simulink model "es2s"  (R2020b)
settings: Solver=VariableStepAuto  StartTime=0.0  StopTime=20  MaxStep=0.001  RelTol=1e-3
values from neighbouring files (symbols this model uses):
  c = 0    [ex 5 residual solution.m]
  k = 100    [ex 5 residual solution.m]
  m = 2    [ex 5 residual solution.m]
undefined symbols (not defined in the file or in its folder): sigbuilder_block
settings Model: Creator=EREN  LastModifiedBy=drart

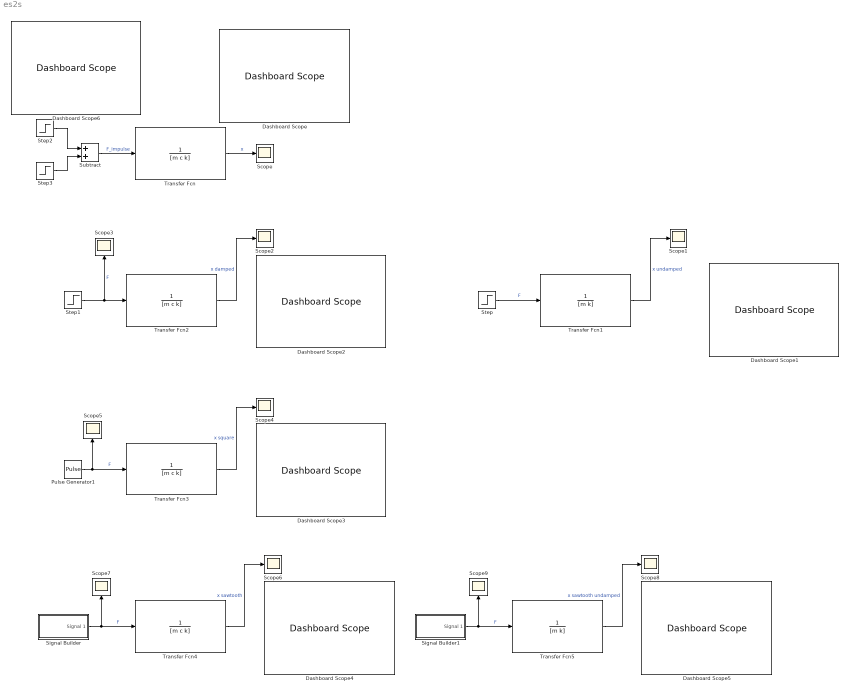
== system es2s ==
  Dashboard Scope{,1..6} (7 alike) : DashboardScope
  Pulse Generator1 : DiscretePulseGenerator  PulseType=Time based  Amplitude=50  Period=100  PulseWidth=5
  Scope{,1..9} (10 alike) : Scope
  Signal Builder : Subsystem  Tag=STV Subsys  LoadFcn=sigbuilder_block('load');  StartFcn=sigbuilder_block('start');  StopFcn=sigbuilder_block('stop');  ClipboardFcn=sigbuilder_block('clipboard');  mask(Sigbuilder block){tuvar=[0:10]}
      mask help: Simulink:masks:SigbuilderBlock_MD
      mask init:
      | if ~strcmp(get_param(bdroot(gcbh),'SimulationStatus'),'stopped') tuvar = sigbuilder_block('maskInit'); end
      settings: CopyFcn=sigbuilder_block('copy');  DeleteFcn=sigbuilder_block('delete');  ModelCloseFcn=sigbuilder_block('modelClose');  PreSaveFcn=sigbuilder_block('preSave');  PauseFcn=sigbuilder_block('pause');  ContinueFcn=sigbuilder_block('continue');  NameChangeFcn=sigbuilder_block('namechange');  OpenFcn=sigbuilder_block('open',[374.4 130.2 550.8 400.2 ]);  CloseFcn=sigbuilder_block('close');
      mask Display: plot(0, 0, 100, 100,[2, 2, 32, 32, 2], [68, 8, 8, 68, 68],[32, 2], [38, 38], [32, 19, 2],[53, 60, 44], [32, 17, 17, 2],[16, 16, 31, 31]);txt = getActiveGroup(gcbh);text(2, 100, txt,'verticalAlignment', 'top');
  Signal Builder1 : Subsystem  Tag=STV Subsys  LoadFcn=sigbuilder_block('load');  StartFcn=sigbuilder_block('start');  StopFcn=sigbuilder_block('stop');  ClipboardFcn=sigbuilder_block('clipboard');  mask(Sigbuilder block){tuvar=[0:10]}
      mask help: Simulink:masks:SigbuilderBlock_MD
      mask init:
      | if ~strcmp(get_param(bdroot(gcbh),'SimulationStatus'),'stopped') tuvar = sigbuilder_block('maskInit'); end
      settings: CopyFcn=sigbuilder_block('copy');  DeleteFcn=sigbuilder_block('delete');  ModelCloseFcn=sigbuilder_block('modelClose');  PreSaveFcn=sigbuilder_block('preSave');  PauseFcn=sigbuilder_block('pause');  ContinueFcn=sigbuilder_block('continue');  NameChangeFcn=sigbuilder_block('namechange');  OpenFcn=sigbuilder_block('open',[374.4 130.2 550.8 400.2 ]);  CloseFcn=sigbuilder_block('close');
      mask Display: plot(0, 0, 100, 100,[2, 2, 32, 32, 2], [68, 8, 8, 68, 68],[32, 2], [38, 38], [32, 19, 2],[53, 60, 44], [32, 17, 17, 2],[16, 16, 31, 31]);txt = getActiveGroup(gcbh);text(2, 100, txt,'verticalAlignment', 'top');
  Step : Step  Time=0  After=1000  SampleTime=0
  Step1 : Step  Time=0  After=1000  SampleTime=0
  Step2 : Step  Time=0  SampleTime=0
  Step3 : Step  Time=0.1  After=-1  SampleTime=0
  Subtract : Sum
  Transfer Fcn{,2..4} (4 alike) : TransferFcn  Denominator=[m c k]
  Transfer Fcn1 : TransferFcn  Denominator=[m k]
  Transfer Fcn5 : TransferFcn  Denominator=[m k]
  wires:
  Transfer Fcn/1 -> Scope/1  "x"
  Subtract/1 -> Transfer Fcn/1  "F_impulse"
  Step/1 -> Transfer Fcn1/1  "F"
  Transfer Fcn1/1 -> Scope1/1  "x undamped"
  Transfer Fcn2/1 -> Scope2/1  "x damped"
  Step1/1 -> Scope3/1, Transfer Fcn2/1  "F"
  Pulse Generator1/1 -> Scope5/1, Transfer Fcn3/1  "F"
  Transfer Fcn3/1 -> Scope4/1  "x square"
  Transfer Fcn4/1 -> Scope6/1  "x sawtooth"
  Signal Builder/1(Signal 1) -> Transfer Fcn4/1, Scope7/1  "F"
  Signal Builder1/1(Signal 1) -> Scope9/1, Transfer Fcn5/1  "F"
  Transfer Fcn5/1 -> Scope8/1  "x sawtooth undamped"
  Step2/1 -> Subtract/1
  Step3/1 -> Subtract/2

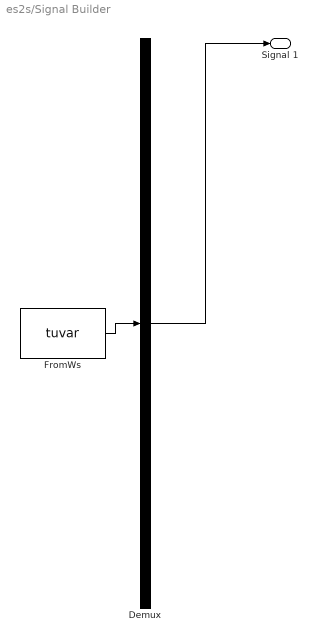
== system es2s/Signal Builder ==
  Demux : Demux  Tag=STV Demux  Outputs=1
      settings: DisplayOption=none
  FromWs : FromWorkspace  Tag=STV FromWs  VariableName=tuvar
      SigBuilderData=|
      | common.afterFinalStr = 'Extrapolate'
      | common.sampleTime = 0
      | dataSet.timeRange = [0 10]
      | dataSet.name = 'Group 1'
      | sbobj.Groups.Name = 'Group 1'
      | sbobj.Groups.Signals.Name = 'Signal 1'
      | sbobj.Groups.Signals.XData = [0 5 5 10]
      | sbobj.Groups.Signals.YData = [0 10 0 0]
  Signal 1 : Outport  Tag=STV Outport
  wires:
  Demux/1 -> Signal 1/1
  FromWs/1 -> Demux/1

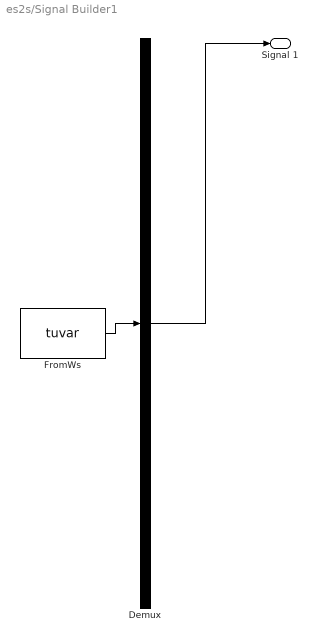
== system es2s/Signal Builder1 ==
  Demux : Demux  Tag=STV Demux  Outputs=1
      settings: DisplayOption=none
  FromWs : FromWorkspace  Tag=STV FromWs  VariableName=tuvar
      SigBuilderData=|
      | common.afterFinalStr = 'Extrapolate'
      | common.sampleTime = 0
      | dataSet.timeRange = [0 10]
      | dataSet.name = 'Group 1'
      | sbobj.Groups.Name = 'Group 1'
      | sbobj.Groups.Signals.Name = 'Signal 1'
      | sbobj.Groups.Signals.XData = [0 5 5 10]
      | sbobj.Groups.Signals.YData = [0 10 0 0]
  Signal 1 : Outport  Tag=STV Outport
  wires:
  FromWs/1 -> Demux/1
  Demux/1 -> Signal 1/1
